simulink model "DeffPrac"  (R2020b)
settings: Solver=VariableStepAuto  StartTime=0.0  StopTime=10  RelTol=1e-3
settings Model: Creator=99003759  LastModifiedBy=99003778

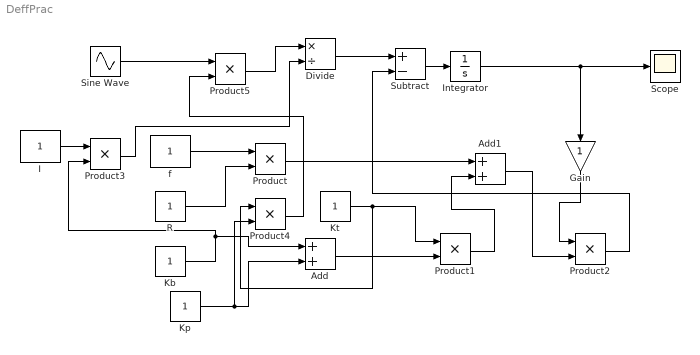
== system DeffPrac ==
  Add : Sum
  Add1 : Sum
  Divide : Product  Inputs=*/
  Gain : Gain
  I : Constant
  Integrator : Integrator
  Kb : Constant
  Kp : Constant
  Kt : Constant
  Product{,1..5} (6 alike) : Product
  R : Constant
  Scope : Scope
  Sine Wave : Sin  SampleTime=0
  Subtract : Sum  Inputs=+-
  f : Constant
  wires:
  Integrator/1 -> Scope/1, Gain/1
  f/1 -> Product/1
  R/1 -> Product/2
  Kb/1 -> Product3/2, Add/1
  Kp/1 -> Product4/2, Add/2
  Kt/1 -> Product4/1, Product1/1
  Add/1 -> Product1/2
  Product/1 -> Add1/1
  Product1/1 -> Add1/2
  Gain/1 -> Product2/1
  Add1/1 -> Product2/2
  I/1 -> Product3/1
  Sine Wave/1 -> Product5/1
  Product4/1 -> Product5/2
  Product5/1 -> Divide/1
  Divide/1 -> Subtract/1
  Product3/1 -> Divide/2
  Product2/1 -> Subtract/2
  Subtract/1 -> Integrator/1
